simulink model "ES320A_MotDrvDiagc"  (R2013b)
settings: Solver=FixedStepDiscrete  StartTime=0.0  StopTime=1  FixedStep=.002  RelTol=1e-3
undefined symbols (not defined in the file): ARCHGLBPRM_2MILLISEC_SEC_F32, MotDrvDiagcErrFilFrq, MotDrvDiagcErrOffs, MotDrvDiagcErrThd, NtcNr1, NtcSts1, PHAONTISUMMAX_NANOSEC_U32, SysSt1
libraries: simulink x23, Fil x12, NxtrAbslt x6, NxtrLim x6
(part 1 of 3)
settings Model: Creator=PallavG  LastModifiedBy=FZG88Y
settings DataIOCC: LimitDataPoints=off  SaveFormat=Structure  ReturnWorkspaceOutputs=on
settings OptimizationCC: BlockReduction=off  InlineParams=on  ZeroExternalMemoryAtStartup=off  ZeroInternalMemoryAtStartup=off  OptimizeModelRefInitCode=on  LifeSpan=1
settings DebuggingCC: SignalInfNanChecking=error  SignalRangeChecking=warning  UnderspecifiedInitializationDetection=Simplified  SolverPrmCheckMsg=error  InheritedTsInSrcMsg=error  DiscreteInheritContinuousMsg=error  SingleTaskRateTransMsg=error  TasksWithSamePriorityMsg=error  SigSpecEnsureSampleTimeMsg=error  CheckMatrixSingularityMsg=error  IntegerOverflowMsg=error  ParameterUnderflowMsg=error  ParameterPrecisionLossMsg=error  ParameterTunabilityLossMsg=error  FixptConstUnderflowMsg=warning  FixptConstOverflowMsg=warning  VectorMatrixConversionMsg=error  SignalLabelMismatchMsg=error  UnconnectedInputMsg=error  UnconnectedOutputMsg=error  UnconnectedLineMsg=error  SFcnCompatibilityMsg=error  UniqueDataStoreMsg=warning  BusObjectLabelMismatch=error  RootOutportRequireBusObject=error  AssertControl=DisableAll  ModelReferenceIOMsg=error  ModelReferenceVersionMismatchMessage=warning  ModelReferenceIOMismatchMessage=error  ModelReferenceCSMismatchMessage=warning  ModelReferenceDataLoggingMessage=error  StateNameClashWarn=warning  StrictBusMsg=ErrorOnBusTreatedAsVector  NonBusSignalsTreatedAsBus=error  SFUnexpectedBacktrackingDiag=error  SFInvalidInputDataAccessInChartInitDiag=error  SFNoUnconditionalDefaultTransitionDiag=error  SFTransitionOutsideNaturalParentDiag=error  SFUnconditionalTransitionShadowingDiag=error  SFUndirectedBroadcastEventsDiag=error
settings ModelReferenceCC: ModelReferenceNumInstancesAllowed=Single
settings RTWCC: SystemTargetFile=autosar.tlc  GenCodeOnly=on  TemplateMakefile=ert_default_tmf  Description=AUTOSAR  GenerateReport=on  ProcessScript=autosar_make_rtw_hook  LaunchReport=on
settings CodeAppCC: GenerateComments=off  IgnoreCustomStorageClasses=off  CustomSymbolStrType=$N$R$M  CustomSymbolStrBlkIO=$N$M  SimulinkBlockComments=off
settings STFCustomTargetCC: ParMdlRefBuildCompliant=on  CompOptLevelCompliant=on  IncludeMdlTerminateFcn=off  CombineOutputUpdateFcns=on  SuppressErrorStatus=on  ERTFirstTimeCompliant=on  ERTCustomFileBanners=on  SupportNonFinite=off  SupportComplex=off  SupportContinuousTime=off  SupportNonInlinedSFcns=off  MATLABClassNameForMDSCustomization=Simulink.SoftwareTarget.ERTCustomization  AutosarCompliant=on  GRTInterface=off  SystemTargetFile=autosar.tlc
settings ERTTargetCC: CodeReplacementLibrary=ANSI_C  ConcurrentExecutionCompliant=off  IncludeMdlTerminateFcn=off  SuppressErrorStatus=on  SupportNonFinite=off  SupportComplex=off  ModelStepFunctionPrototypeControlCompliant=off  CPPClassGenCompliant=off  AutosarCompliant=on  InlinedParameterPlacement=NonHierarchical  ERTCustomFileTemplate=example_file_process.tlc  EnableUserReplacementTypes=on

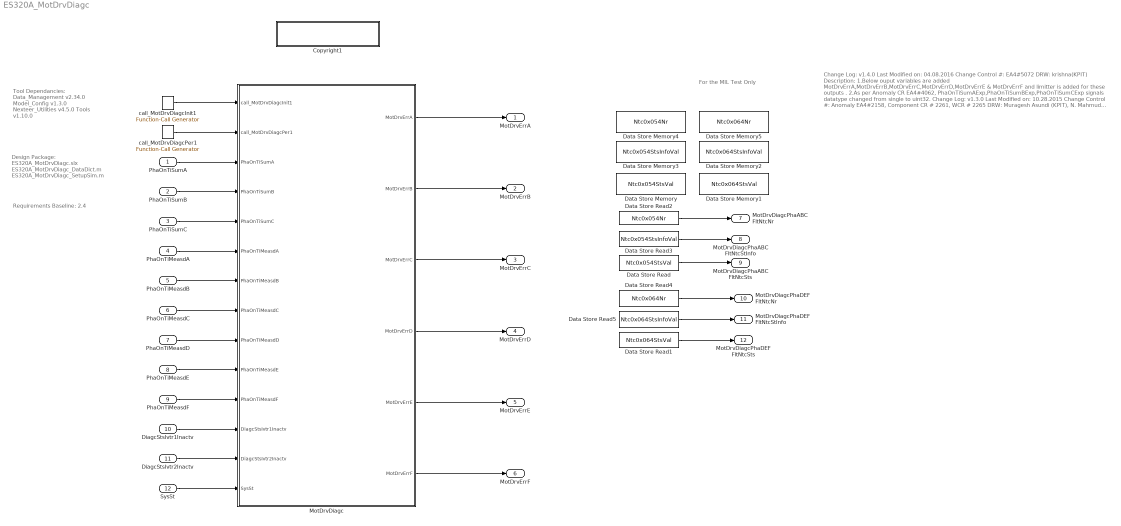
== system ES320A_MotDrvDiagc ==
  note: For the MIL Test Only
  note: Requirements Baseline: 2.4
  note: Design Package:
      | ES320A_MotDrvDiagc.slx
      | ES320A_MotDrvDiagc_DataDict.m
      | ES320A_MotDrvDiagc_SetupSim.m
  note: Change Log:  v1.4.0
      | Last Modified on: 04.08.2016
      | Change Control #: EA4#5072
      | DRW: krishna(KPIT)
      | Description:
      | 1.Below ouput variables are added
      |   MotDrvErrA,MotDrvErrB,MotDrvErrC,MotDrvErrD,MotDrvErrE & MotDrvErrF
      |   and limitter is added for these outputs .
      | 2.As per Anomaly CR EA4#4062, PhaOnTiSumAExp,PhaOnTiSumBExp,PhaOnTiSumCExp signals datatype
      | changed from single to uint32.
      |
      | Change Log:  v1.3.0
      | Last Modified on: 10.28.2015
      | Change Control #: Anomaly EA4#2158, Component CR # 2261, WCR # 2265
      | DRW:  Muragesh Asundi (KPIT), N. Mahmud
      | Description:
      | - Anomaly 2158 is fixed
      | - Also fixes the logic for setting the prepass, prefail for NTC54, 64
      |
      | Change Log:  v1.2.0
      | Last Modified on: 09.30.2015
      | Change Control #: Anomaly EA4#1595, Component CR # 1763, WCR # 1768
      | DRW:  N. Mahmud
      | Description:
      | - Anomaly 1595 is fixed
      |
      | Change Log:  v1.1.0
      | Date: 21-Aug-2015
      | Change Control #: EA4#1383
      | DRW:  Muragesh Asundi
      | Description:
      | - 'MotCtrl' prefix removed from Inputs.
      | - Global constant 'ARCHGLBPRM_2MILLISEC_SEC_F32' used
      |
      | Change Log:  v1.0.0
      | Date: 12-Aug-2015
      | Change Control #: EA4#1004
      | DRW:  Pallav Garg
      | Description:
      | - Initial Release of EA4 1.0.0
  note: Tool Dependancies:
      |
      | Data_Management v2.34.0
      | Model_Config v1.3.0
      | Nexteer_Utilities v4.5.0
      | Tools v1.10.0
  PhaOnTiSumA : Inport  RequirementInfo={'linktype_rmi_doors' '0000cf4c (/ESG Group/FDD Module Requirements/EA4 Specific/ES320A_MotDrvDiagc)' '#ES320A_92' 'true' 'REQ: ES320A_92' '' } %GIDa_5596e1da_8470_45ec_add7_471382801404
  PhaOnTiSumB : Inport  RequirementInfo={'linktype_rmi_doors' '0000cf4c (/ESG Group/FDD Module Requirements/EA4 Specific/ES320A_MotDrvDiagc)' '#ES320A_181' 'true' 'REQ: ES320A_181' '' } %GIDa_210e4004_e252_48ab_913f_51028c960f64  Port=2
  PhaOnTiSumC : Inport  RequirementInfo={'linktype_rmi_doors' '0000cf4c (/ESG Group/FDD Module Requirements/EA4 Specific/ES320A_MotDrvDiagc)' '#ES320A_180' 'true' 'REQ: ES320A_180' '' } %GIDa_70180edb_7662_4ea3_bdb5_76072d466fb3  Port=3
  PhaOnTiMeasdA : Inport  RequirementInfo={'linktype_rmi_doors' '0000cf4c (/ESG Group/FDD Module Requirements/EA4 Specific/ES320A_MotDrvDiagc)' '#ES320A_93' 'true' 'REQ: ES320A_93' '' } %GIDa_afd0493b_6092_46df_9f0f_5569d48d5c6b  Port=4
  PhaOnTiMeasdB : Inport  RequirementInfo={'linktype_rmi_doors' '0000cf4c (/ESG Group/FDD Module Requirements/EA4 Specific/ES320A_MotDrvDiagc)' '#ES320A_183' 'true' 'REQ: ES320A_183' '' } %GIDa_f1d745cb_f7fe_4c90_af22_8ff78fec897d  Port=5
  PhaOnTiMeasdC : Inport  RequirementInfo={'linktype_rmi_doors' '0000cf4c (/ESG Group/FDD Module Requirements/EA4 Specific/ES320A_MotDrvDiagc)' '#ES320A_182' 'true' 'REQ: ES320A_182' '' } %GIDa_39f5c4e7_f024_452a_b628_18bd5ec5a4db  Port=6
  PhaOnTiMeasdD : Inport  RequirementInfo={'linktype_rmi_doors' '0000cf4c (/ESG Group/FDD Module Requirements/EA4 Specific/ES320A_MotDrvDiagc)' '#ES320A_186' 'true' 'REQ: ES320A_186' '' } %GIDa_d08ff034_005a_421c_9828_e45c8ccc9891  Port=7
  PhaOnTiMeasdE : Inport  RequirementInfo={'linktype_rmi_doors' '0000cf4c (/ESG Group/FDD Module Requirements/EA4 Specific/ES320A_MotDrvDiagc)' '#ES320A_185' 'true' 'REQ: ES320A_185' '' } %GIDa_b8a159d2_0664_4d31_91d9_6025fe5fa159  Port=8
  PhaOnTiMeasdF : Inport  RequirementInfo={'linktype_rmi_doors' '0000cf4c (/ESG Group/FDD Module Requirements/EA4 Specific/ES320A_MotDrvDiagc)' '#ES320A_184' 'true' 'REQ: ES320A_184' '' } %GIDa_0e7ed425_9747_4174_868c_b8b73984cdca  Port=9
  DiagcStsIvtr1Inactv : Inport  RequirementInfo={'linktype_rmi_doors' '0000cf4c (/ESG Group/FDD Module Requirements/EA4 Specific/ES320A_MotDrvDiagc)' '#ES320A_187' 'true' 'REQ: ES320A_187' '' } %GIDa_a171dc8c_548f_4e98_b628_0ce941fa05d6  Port=10
  DiagcStsIvtr2Inactv : Inport  RequirementInfo={'linktype_rmi_doors' '0000cf4c (/ESG Group/FDD Module Requirements/EA4 Specific/ES320A_MotDrvDiagc)' '#ES320A_189' 'true' 'REQ: ES320A_189' '' } %GIDa_3630ab79_1ac9_45bf_b99f_436db09e5141  Port=11
  SysSt : Inport  RequirementInfo={'linktype_rmi_doors' '0000cf4c (/ESG Group/FDD Module Requirements/EA4 Specific/ES320A_MotDrvDiagc)' '#ES320A_188' 'true' 'REQ: ES320A_188' '' } %GIDa_0e538df3_d78e_40dd_9cd2_699620956152  Port=12
  Copyright1 : Subsystem  Description=|  RequirementInfo={} %GIDa_31a5e494_f362_4315_ad68_df9135c8582b  mask(Copyright Information){none=on}
      | Copyright info block.                                               
      |                                                                     
      | Place copyright information at the top of every subsystem in design.
      mask prompts: none "No parameters"
      mask help: Place copyright information at the top of every subsystem in design.
      mask Display:
      | NxtrConf = 'Nexteer Confidential';
      | 
      | sys = bdroot; %handle for the current model ("system")
      | first = get_param(sys,'Created');
      | if(isempty(first))
      |     first = datestr(now,'yyyy');
      | else
      |     first = first(end-3:end);  %year is last four digits
      | end
      | 
      | last = get_param(sys,'LastModifiedDate');
      | if isempty(last)
      |     last = datestr(now,'yyyy');
      | else
      |     last = last(end-3:end);
      | end
      | 
      | if strcmp(first,last)
      |     fprintf('%s\nCopyright  %s Nexteer',NxtrConf,first);
      | else
      |     fprintf('%s\n%s%s-%s Nexteer',NxtrConf,char(169),first,last);
      | end
  Data Store Read : DataStoreRead  DataStoreName=Ntc0x054StsVal  SampleTime=.002
  Data Store Read1 : DataStoreRead  DataStoreName=Ntc0x064StsVal  SampleTime=.002
  Data Store Read2 : DataStoreRead  DataStoreName=Ntc0x054Nr  SampleTime=.002
  Data Store Read3 : DataStoreRead  DataStoreName=Ntc0x054StsInfoVal  SampleTime=.002
  Data Store Read4 : DataStoreRead  DataStoreName=Ntc0x064Nr  SampleTime=.002
  Data Store Read5 : DataStoreRead  DataStoreName=Ntc0x064StsInfoVal  SampleTime=.002
  Data Store Memory : DataStoreMemory  DataStoreName=Ntc0x054StsVal  ReadBeforeWriteMsg=warning  WriteAfterWriteMsg=warning  WriteAfterReadMsg=warning  InitialValue=NtcSts1.NTCSTS_PASSD
  Data Store Memory1 : DataStoreMemory  DataStoreName=Ntc0x064StsVal  ReadBeforeWriteMsg=warning  WriteAfterWriteMsg=warning  WriteAfterReadMsg=warning  InitialValue=NtcSts1.NTCSTS_PASSD
  Data Store Memory2 : DataStoreMemory  DataStoreName=Ntc0x064StsInfoVal  ReadBeforeWriteMsg=warning  WriteAfterWriteMsg=warning  WriteAfterReadMsg=warning
  Data Store Memory3 : DataStoreMemory  DataStoreName=Ntc0x054StsInfoVal  ReadBeforeWriteMsg=warning  WriteAfterWriteMsg=warning  WriteAfterReadMsg=warning
  Data Store Memory4 : DataStoreMemory  DataStoreName=Ntc0x054Nr  ReadBeforeWriteMsg=warning  WriteAfterWriteMsg=warning  WriteAfterReadMsg=warning  InitialValue=NtcNr1.NTCNR_0X054
  Data Store Memory5 : DataStoreMemory  DataStoreName=Ntc0x064Nr  ReadBeforeWriteMsg=warning  WriteAfterWriteMsg=warning  WriteAfterReadMsg=warning  InitialValue=NtcNr1.NTCNR_0X064
  MotDrvDiagc : Subsystem
  call_MotDrvDiagcInit1 : simulink/Ports & Subsystems/Function-Call Generator  sample_time=.002  numberOfIterations=1
  call_MotDrvDiagcPer1 : simulink/Ports & Subsystems/Function-Call Generator  sample_time=.002  numberOfIterations=1
  MotDrvErrA : Outport
  MotDrvErrB : Outport  Port=2
  MotDrvErrC : Outport  Port=3
  MotDrvErrD : Outport  Port=4
  MotDrvErrE : Outport  Port=5
  MotDrvErrF : Outport  Port=6
  MotDrvDiagcPhaABCFltNtcNr : Outport  Port=7
  MotDrvDiagcPhaABCFltNtcStInfo : Outport  Port=8
  MotDrvDiagcPhaABCFltNtcSts : Outport  Port=9
  MotDrvDiagcPhaDEFFltNtcNr : Outport  Port=10
  MotDrvDiagcPhaDEFFltNtcStInfo : Outport  Port=11
  MotDrvDiagcPhaDEFFltNtcSts : Outport  Port=12
  wires:
  PhaOnTiSumA/1 -> MotDrvDiagc/3(PhaOnTiSumA)
  PhaOnTiSumB/1 -> MotDrvDiagc/4(PhaOnTiSumB)
  PhaOnTiSumC/1 -> MotDrvDiagc/5(PhaOnTiSumC)
  PhaOnTiMeasdA/1 -> MotDrvDiagc/6(PhaOnTiMeasdA)
  PhaOnTiMeasdB/1 -> MotDrvDiagc/7(PhaOnTiMeasdB)
  PhaOnTiMeasdC/1 -> MotDrvDiagc/8(PhaOnTiMeasdC)
  PhaOnTiMeasdD/1 -> MotDrvDiagc/9(PhaOnTiMeasdD)
  PhaOnTiMeasdE/1 -> MotDrvDiagc/10(PhaOnTiMeasdE)
  PhaOnTiMeasdF/1 -> MotDrvDiagc/11(PhaOnTiMeasdF)
  DiagcStsIvtr1Inactv/1 -> MotDrvDiagc/12(DiagcStsIvtr1Inactv)
  DiagcStsIvtr2Inactv/1 -> MotDrvDiagc/13(DiagcStsIvtr2Inactv)
  call_MotDrvDiagcPer1/1 -> MotDrvDiagc/2(call_MotDrvDiagcPer1)
  SysSt/1 -> MotDrvDiagc/14(SysSt)
  call_MotDrvDiagcInit1/1 -> MotDrvDiagc/1(call_MotDrvDiagcInit1)
  Data Store Read/1 -> MotDrvDiagcPhaABCFltNtcSts/1
  Data Store Read1/1 -> MotDrvDiagcPhaDEFFltNtcSts/1
  Data Store Read2/1 -> MotDrvDiagcPhaABCFltNtcNr/1
  Data Store Read3/1 -> MotDrvDiagcPhaABCFltNtcStInfo/1
  Data Store Read4/1 -> MotDrvDiagcPhaDEFFltNtcNr/1
  Data Store Read5/1 -> MotDrvDiagcPhaDEFFltNtcStInfo/1
  MotDrvDiagc/1(MotDrvErrA) -> MotDrvErrA/1
  MotDrvDiagc/2(MotDrvErrB) -> MotDrvErrB/1
  MotDrvDiagc/3(MotDrvErrC) -> MotDrvErrC/1
  MotDrvDiagc/6(MotDrvErrF) -> MotDrvErrF/1
  MotDrvDiagc/5(MotDrvErrE) -> MotDrvErrE/1
  MotDrvDiagc/4(MotDrvErrD) -> MotDrvErrD/1

== system ES320A_MotDrvDiagc/Copyright1 ==

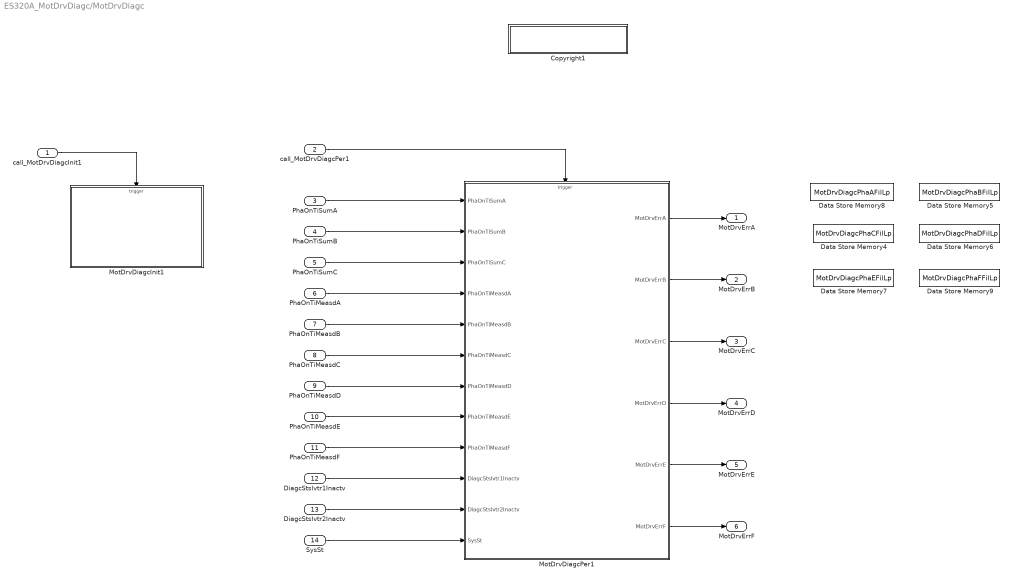
== system ES320A_MotDrvDiagc/MotDrvDiagc ==
  call_MotDrvDiagcInit1 : Inport
  call_MotDrvDiagcPer1 : Inport  Port=2
  PhaOnTiSumA : Inport  RequirementInfo={} %GIDa_46cfb15b_79f9_4df3_959a_549c348c89d2  Port=3
  PhaOnTiSumB : Inport  RequirementInfo="{}  %GIDa_e4750f2c_32c2_4abf_a78a_5be133e16fa3"  Port=4
  PhaOnTiSumC : Inport  Port=5
  PhaOnTiMeasdA : Inport  Port=6
  PhaOnTiMeasdB : Inport  Port=7
  PhaOnTiMeasdC : Inport  Port=8
  PhaOnTiMeasdD : Inport  Port=9
  PhaOnTiMeasdE : Inport  Port=10
  PhaOnTiMeasdF : Inport  Port=11
  DiagcStsIvtr1Inactv : Inport  Port=12
  DiagcStsIvtr2Inactv : Inport  Port=13
  SysSt : Inport  Port=14
  Copyright1 : Subsystem  Description=|  RequirementInfo={} %GIDa_40b2bef5_baed_40e1_9760_ec08ea904b84  mask(Copyright Information){none=on}
      | Copyright info block.                                               
      |                                                                     
      | Place copyright information at the top of every subsystem in design.
      mask prompts: none "No parameters"
      mask help: Place copyright information at the top of every subsystem in design.
      mask Display:
      | NxtrConf = 'Nexteer Confidential';
      | 
      | sys = bdroot; %handle for the current model ("system")
      | first = get_param(sys,'Created');
      | if(isempty(first))
      |     first = datestr(now,'yyyy');
      | else
      |     first = first(end-3:end);  %year is last four digits
      | end
      | 
      | last = get_param(sys,'LastModifiedDate');
      | if isempty(last)
      |     last = datestr(now,'yyyy');
      | else
      |     last = last(end-3:end);
      | end
      | 
      | if strcmp(first,last)
      |     fprintf('%s\nCopyright  %s Nexteer',NxtrConf,first);
      | else
      |     fprintf('%s\n%s%s-%s Nexteer',NxtrConf,char(169),first,last);
      | end
  Data Store Memory4 : DataStoreMemory  DataStoreName=MotDrvDiagcPhaCFilLp  InitialValue=struct('FilSt',single(0),'FilGain',single(0))  OutDataTypeStr=Bus: FilLpRec1  StateMustResolveToSignalObject=on
  Data Store Memory5 : DataStoreMemory  DataStoreName=MotDrvDiagcPhaBFilLp  InitialValue=struct('FilSt',single(0),'FilGain',single(0))  OutDataTypeStr=Bus: FilLpRec1  StateMustResolveToSignalObject=on
  Data Store Memory6 : DataStoreMemory  DataStoreName=MotDrvDiagcPhaDFilLp  InitialValue=struct('FilSt',single(0),'FilGain',single(0))  OutDataTypeStr=Bus: FilLpRec1  StateMustResolveToSignalObject=on
  Data Store Memory7 : DataStoreMemory  DataStoreName=MotDrvDiagcPhaEFilLp  InitialValue=struct('FilSt',single(0),'FilGain',single(0))  OutDataTypeStr=Bus: FilLpRec1  StateMustResolveToSignalObject=on
  Data Store Memory8 : DataStoreMemory  DataStoreName=MotDrvDiagcPhaAFilLp  InitialValue=struct('FilSt',single(0),'FilGain',single(0))  OutDataTypeStr=Bus: FilLpRec1  StateMustResolveToSignalObject=on
  Data Store Memory9 : DataStoreMemory  DataStoreName=MotDrvDiagcPhaFFilLp  InitialValue=struct('FilSt',single(0),'FilGain',single(0))  OutDataTypeStr=Bus: FilLpRec1  StateMustResolveToSignalObject=on
  MotDrvDiagcInit1 : Subsystem
  MotDrvDiagcPer1 : Subsystem  RequirementInfo={'linktype_rmi_doors' '0000cf4c (/ESG Group/FDD Module Requirements/EA4 Specific/ES320A_MotDrvDiagc)' '#ES320A_158' 'true' 'REQ: ES320A_158' '' ; 'linktype_rmi_doors' '0000cf4c (/ESG Group/FDD Module Requirements/EA4 Specific/ES320A_MotDrvDiagc)' '#ES320A_160' 'true' 'REQ: ES320A_160' '' } %GIDa_e8681813_4efe_4d27_b36c_1f578861e450
  MotDrvErrA : Outport  RequirementInfo={'linktype_rmi_doors' '0000cf4c (/ESG Group/FDD Module Requirements/EA4 Specific/ES320A_MotDrvDiagc)' '#ES320A_207' 'true' 'REQ: ES320A_207' '' } %GIDa_9503e4c0_a7fc_485b_98a2_972c7f7bfe08
  MotDrvErrB : Outport  RequirementInfo={'linktype_rmi_doors' '0000cf4c (/ESG Group/FDD Module Requirements/EA4 Specific/ES320A_MotDrvDiagc)' '#ES320A_207' 'true' 'REQ: ES320A_207' '' } %GIDa_84eb9338_eb0d_4322_a092_261cb67f10b3  Port=2
  MotDrvErrC : Outport  RequirementInfo={'linktype_rmi_doors' '0000cf4c (/ESG Group/FDD Module Requirements/EA4 Specific/ES320A_MotDrvDiagc)' '#ES320A_206' 'true' 'REQ: ES320A_206' '' } %GIDa_9cdd7cca_5e7a_4907_9b10_5ffe4d089f88  Port=3
  MotDrvErrD : Outport  RequirementInfo={'linktype_rmi_doors' '0000cf4c (/ESG Group/FDD Module Requirements/EA4 Specific/ES320A_MotDrvDiagc)' '#ES320A_205' 'true' 'REQ: ES320A_205' '' } %GIDa_f1a02c70_5322_40ef_93da_787d66763215  Port=4
  MotDrvErrE : Outport  RequirementInfo={'linktype_rmi_doors' '0000cf4c (/ESG Group/FDD Module Requirements/EA4 Specific/ES320A_MotDrvDiagc)' '#ES320A_204' 'true' 'REQ: ES320A_204' '' } %GIDa_72a22f43_ae99_4136_a3a8_5e5738f24507  Port=5
  MotDrvErrF : Outport  RequirementInfo={'linktype_rmi_doors' '0000cf4c (/ESG Group/FDD Module Requirements/EA4 Specific/ES320A_MotDrvDiagc)' '#ES320A_203' 'true' 'REQ: ES320A_203' '' } %GIDa_ddfd7e60_4b6a_46f1_bcfa_2573913685dc  Port=6
  wires:
  PhaOnTiMeasdC/1 -> MotDrvDiagcPer1/6(PhaOnTiMeasdC)
  PhaOnTiMeasdD/1 -> MotDrvDiagcPer1/7(PhaOnTiMeasdD)
  PhaOnTiSumB/1 -> MotDrvDiagcPer1/2(PhaOnTiSumB)
  PhaOnTiMeasdE/1 -> MotDrvDiagcPer1/8(PhaOnTiMeasdE)
  PhaOnTiMeasdF/1 -> MotDrvDiagcPer1/9(PhaOnTiMeasdF)
  PhaOnTiSumC/1 -> MotDrvDiagcPer1/3(PhaOnTiSumC)
  DiagcStsIvtr1Inactv/1 -> MotDrvDiagcPer1/10(DiagcStsIvtr1Inactv)
  DiagcStsIvtr2Inactv/1 -> MotDrvDiagcPer1/11(DiagcStsIvtr2Inactv)
  call_MotDrvDiagcPer1/1 -> MotDrvDiagcPer1/Trigger
  SysSt/1 -> MotDrvDiagcPer1/12(SysSt)
  call_MotDrvDiagcInit1/1 -> MotDrvDiagcInit1/Trigger
  PhaOnTiSumA/1 -> MotDrvDiagcPer1/1(PhaOnTiSumA)
  MotDrvDiagcPer1/1(MotDrvErrA) -> MotDrvErrA/1
  MotDrvDiagcPer1/2(MotDrvErrB) -> MotDrvErrB/1
  MotDrvDiagcPer1/3(MotDrvErrC) -> MotDrvErrC/1
  MotDrvDiagcPer1/4(MotDrvErrD) -> MotDrvErrD/1
  MotDrvDiagcPer1/5(MotDrvErrE) -> MotDrvErrE/1
  MotDrvDiagcPer1/6(MotDrvErrF) -> MotDrvErrF/1
  PhaOnTiMeasdA/1 -> MotDrvDiagcPer1/4(PhaOnTiMeasdA)
  PhaOnTiMeasdB/1 -> MotDrvDiagcPer1/5(PhaOnTiMeasdB)

== system ES320A_MotDrvDiagc/MotDrvDiagc/Copyright1 ==

== system ES320A_MotDrvDiagc/MotDrvDiagc/MotDrvDiagcInit1 ==
  function : TriggerPort  TriggerType=function-call
  Copyright1 : Subsystem  Description=|  RequirementInfo={} %GIDa_0a1cd7fa_88a7_493f_9ffa_3855db88fd16  mask(Copyright Information){none=on}
      | Copyright info block.                                               
      |                                                                     
      | Place copyright information at the top of every subsystem in design.
      mask prompts: none "No parameters"
      mask help: Place copyright information at the top of every subsystem in design.
      mask Display:
      | NxtrConf = 'Nexteer Confidential';
      | 
      | sys = bdroot; %handle for the current model ("system")
      | first = get_param(sys,'Created');
      | if(isempty(first))
      |     first = datestr(now,'yyyy');
      | else
      |     first = first(end-3:end);  %year is last four digits
      | end
      | 
      | last = get_param(sys,'LastModifiedDate');
      | if isempty(last)
      |     last = datestr(now,'yyyy');
      | else
      |     last = last(end-3:end);
      | end
      | 
      | if strcmp(first,last)
      |     fprintf('%s\nCopyright  %s Nexteer',NxtrConf,first);
      | else
      |     fprintf('%s\n%s%s-%s Nexteer',NxtrConf,char(169),first,last);
      | end
  MotDrvDiagcPhaAFilLpInit : Fil/FilLpInit  Ic=0  Ts=ARCHGLBPRM_2MILLISEC_SEC_F32  Freq=MotDrvDiagcErrFilFrq  StVar=MotDrvDiagcPhaAFilLp
  MotDrvDiagcPhaBFilLpInit : Fil/FilLpInit  Ic=0  Ts=ARCHGLBPRM_2MILLISEC_SEC_F32  Freq=MotDrvDiagcErrFilFrq  StVar=MotDrvDiagcPhaBFilLp
  MotDrvDiagcPhaCFilLpInit : Fil/FilLpInit  Ic=0  Ts=ARCHGLBPRM_2MILLISEC_SEC_F32  Freq=MotDrvDiagcErrFilFrq  StVar=MotDrvDiagcPhaCFilLp
  MotDrvDiagcPhaDFilLpInit : Fil/FilLpInit  Ic=0  Ts=ARCHGLBPRM_2MILLISEC_SEC_F32  Freq=MotDrvDiagcErrFilFrq  StVar=MotDrvDiagcPhaDFilLp
  MotDrvDiagcPhaEFilLpInit : Subsystem  AncestorBlock=Fil/FilLpInit  mask(FilLpInit){Ic=0, Ts=ARCHGLBPRM_2MILLISEC_SEC_F32, Freq=MotDrvDiagcErrFilFrq, StVar=MotDrvDiagcPhaEFilLp}
      mask prompts: Ic "Initial Value"; Ts "TimeStep:"; Freq "Frequency:"; StVar "State Variable"
      mask init:
      | blk = gcb;
      | set_param([blk '/FilLpUpdGain'],'Ts',Ts)
      | set_param([blk '/FilLpUpdGain'],'StVar',StVar)
      | set_param([blk '/Freq'],'Value',Freq)
      | set_param([blk '/Ic'],'Value',Ic)
      | set_param([ blk '/Data Store Write'],'DataStoreName',StVar)
      | try
      |     dt = evalin('base',[StVar '.EngDT']);
      | catch err
      |     if strcmp(err.identifier,'MATLAB:undefinedVarOrClass')
      |         dt = struct.FilLpRec1;
      |     end
      | end
      | if isa(dt,'struct.FilLpRec1')
      | set_param([ blk '/Data Store Write'],'DataStoreElements',[StVar '.FilGain'])
      | elseif isa(dt,'struct.FilHpRec1')
      | set_param([ blk '/Data Store Write'],'DataStoreElements',[StVar '.FilLpRec.FilGain'])
      | else
      |     error('Incorrect data class.');
      | end
      mask Display:
      | text(0.35,0.9,'FilLpInit')
      | text(0.05,0.7,['Ic: ' Ic])
      | text(0.05,0.5,['Ts: ' Ts])
      | text(0.05,0.3,['Freq: ' Freq])
      | text(0.05,0.1,['StVar: ' StVar])
  MotDrvDiagcPhaFFilLpInit : Subsystem  AncestorBlock=Fil/FilLpInit  mask(FilLpInit){Ic=0, Ts=ARCHGLBPRM_2MILLISEC_SEC_F32, Freq=MotDrvDiagcErrFilFrq, StVar=MotDrvDiagcPhaFFilLp}
      mask prompts: Ic "Initial Value"; Ts "TimeStep:"; Freq "Frequency:"; StVar "State Variable"
      mask init: same as ES320A_MotDrvDiagc/MotDrvDiagc/MotDrvDiagcInit1/MotDrvDiagcPhaEFilLpInit
      mask Display:
      | text(0.35,0.9,'FilLpInit')
      | text(0.05,0.7,['Ic: ' Ic])
      | text(0.05,0.5,['Ts: ' Ts])
      | text(0.05,0.3,['Freq: ' Freq])
      | text(0.05,0.1,['StVar: ' StVar])

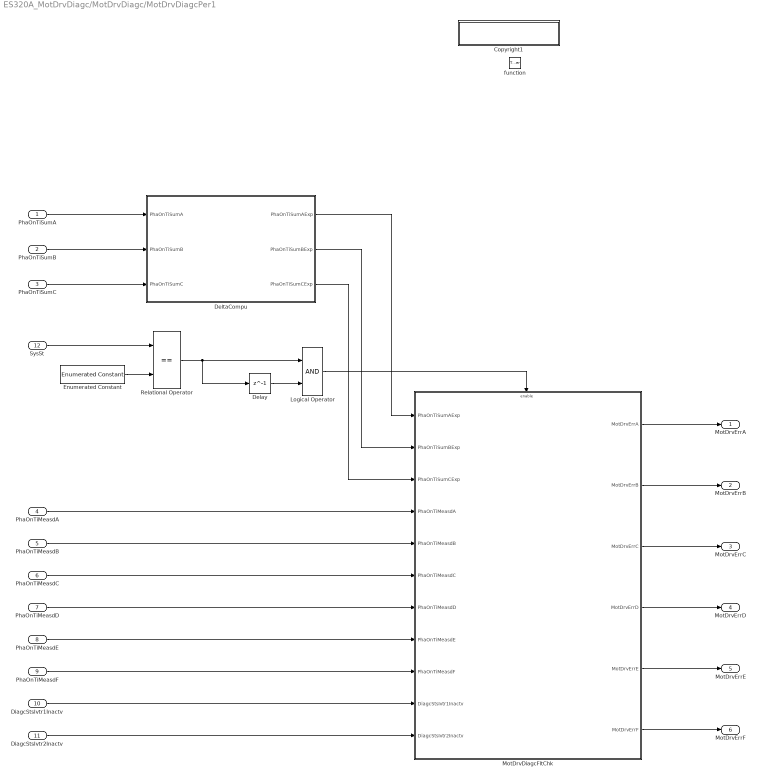
== system ES320A_MotDrvDiagc/MotDrvDiagc/MotDrvDiagcPer1 ==
  PhaOnTiSumA : Inport
  PhaOnTiSumB : Inport  Port=2
  PhaOnTiSumC : Inport  Port=3
  PhaOnTiMeasdA : Inport  Port=4
  PhaOnTiMeasdB : Inport  Port=5
  PhaOnTiMeasdC : Inport  Port=6
  PhaOnTiMeasdD : Inport  Port=7
  PhaOnTiMeasdE : Inport  Port=8
  PhaOnTiMeasdF : Inport  Port=9
  DiagcStsIvtr1Inactv : Inport  Port=10
  DiagcStsIvtr2Inactv : Inport  Port=11
  SysSt : Inport  Port=12  OutDataTypeStr=Enum: SysSt1
  function : TriggerPort  TriggerType=function-call
  Copyright1 : Subsystem  Description=|  RequirementInfo={} %GIDa_b6a8f04b_092f_4b64_aeb7_200da596c9ae  mask(Copyright Information){none=on}
      | Copyright info block.                                               
      |                                                                     
      | Place copyright information at the top of every subsystem in design.
      mask prompts: none "No parameters"
      mask help: Place copyright information at the top of every subsystem in design.
      mask Display:
      | NxtrConf = 'Nexteer Confidential';
      | 
      | sys = bdroot; %handle for the current model ("system")
      | first = get_param(sys,'Created');
      | if(isempty(first))
      |     first = datestr(now,'yyyy');
      | else
      |     first = first(end-3:end);  %year is last four digits
      | end
      | 
      | last = get_param(sys,'LastModifiedDate');
      | if isempty(last)
      |     last = datestr(now,'yyyy');
      | else
      |     last = last(end-3:end);
      | end
      | 
      | if strcmp(first,last)
      |     fprintf('%s\nCopyright  %s Nexteer',NxtrConf,first);
      | else
      |     fprintf('%s\n%s%s-%s Nexteer',NxtrConf,char(169),first,last);
      | end
  Delay : Delay  DelayLength=1  InitialCondition=0  StateName=UnitDly
  DeltaCompu : Subsystem
  Enumerated Constant : simulink/Sources/Enumerated Constant  OutDataTypeStr=Enum: SysSt1  Value=SysSt1.SYSST_ENA  SampleTime=inf
  Logical Operator : Logic  AllPortsSameDT=off  OutDataTypeStr=boolean
  MotDrvDiagcFltChk : Subsystem
  Relational Operator : RelationalOperator  Operator===  OutDataTypeStr=boolean
  MotDrvErrA : Outport
  MotDrvErrB : Outport  Port=2
  MotDrvErrC : Outport  Port=3
  MotDrvErrD : Outport  Port=4
  MotDrvErrE : Outport  Port=5
  MotDrvErrF : Outport  Port=6
  wires:
  PhaOnTiMeasdA/1 -> MotDrvDiagcFltChk/4(PhaOnTiMeasdA)
  PhaOnTiMeasdB/1 -> MotDrvDiagcFltChk/5(PhaOnTiMeasdB)
  PhaOnTiMeasdC/1 -> MotDrvDiagcFltChk/6(PhaOnTiMeasdC)
  PhaOnTiMeasdD/1 -> MotDrvDiagcFltChk/7(PhaOnTiMeasdD)
  PhaOnTiMeasdE/1 -> MotDrvDiagcFltChk/8(PhaOnTiMeasdE)
  PhaOnTiMeasdF/1 -> MotDrvDiagcFltChk/9(PhaOnTiMeasdF)
  DiagcStsIvtr1Inactv/1 -> MotDrvDiagcFltChk/10(DiagcStsIvtr1Inactv)
  DiagcStsIvtr2Inactv/1 -> MotDrvDiagcFltChk/11(DiagcStsIvtr2Inactv)
  Logical Operator/1 -> MotDrvDiagcFltChk/Enable
  SysSt/1 -> Relational Operator/1
  Enumerated Constant/1 -> Relational Operator/2
  PhaOnTiSumC/1 -> DeltaCompu/3(PhaOnTiSumC)
  PhaOnTiSumB/1 -> DeltaCompu/2(PhaOnTiSumB)
  DeltaCompu/1(PhaOnTiSumAExp) -> MotDrvDiagcFltChk/1(PhaOnTiSumAExp)
  DeltaCompu/2(PhaOnTiSumBExp) -> MotDrvDiagcFltChk/2(PhaOnTiSumBExp)
  DeltaCompu/3(PhaOnTiSumCExp) -> MotDrvDiagcFltChk/3(PhaOnTiSumCExp)
  PhaOnTiSumA/1 -> DeltaCompu/1(PhaOnTiSumA)
  Delay/1 -> Logical Operator/2
  Relational Operator/1 -> Delay/1, Logical Operator/1
  MotDrvDiagcFltChk/1(MotDrvErrA) -> MotDrvErrA/1
  MotDrvDiagcFltChk/2(MotDrvErrB) -> MotDrvErrB/1
  MotDrvDiagcFltChk/3(MotDrvErrC) -> MotDrvErrC/1
  MotDrvDiagcFltChk/5(MotDrvErrE) -> MotDrvErrE/1
  MotDrvDiagcFltChk/4(MotDrvErrD) -> MotDrvErrD/1
  MotDrvDiagcFltChk/6(MotDrvErrF) -> MotDrvErrF/1

== system ES320A_MotDrvDiagc/MotDrvDiagc/MotDrvDiagcInit1/Copyright1 ==

== system ES320A_MotDrvDiagc/MotDrvDiagc/MotDrvDiagcInit1/MotDrvDiagcPhaEFilLpInit ==
  Data Store Write : DataStoreWrite  DataStoreName=MotDrvDiagcPhaEFilLp  DataStoreElements=MotDrvDiagcPhaEFilLp.FilGain
  FilLpUpdGain : Fil/FilLpUpdGain  Ts=ARCHGLBPRM_2MILLISEC_SEC_F32  StVar=MotDrvDiagcPhaEFilLp
  Freq : Constant  Value=MotDrvDiagcErrFilFrq  OutDataTypeStr=single
  Ic : Constant  Value=0  OutDataTypeStr=single
  wires:
  Ic/1 -> Data Store Write/1
  Freq/1 -> FilLpUpdGain/1

== system ES320A_MotDrvDiagc/MotDrvDiagc/MotDrvDiagcInit1/MotDrvDiagcPhaFFilLpInit ==
  Data Store Write : DataStoreWrite  DataStoreName=MotDrvDiagcPhaFFilLp  DataStoreElements=MotDrvDiagcPhaFFilLp.FilGain
  FilLpUpdGain : Fil/FilLpUpdGain  Ts=ARCHGLBPRM_2MILLISEC_SEC_F32  StVar=MotDrvDiagcPhaFFilLp
  Freq : Constant  Value=MotDrvDiagcErrFilFrq  OutDataTypeStr=single
  Ic : Constant  Value=0  OutDataTypeStr=single
  wires:
  Ic/1 -> Data Store Write/1
  Freq/1 -> FilLpUpdGain/1

== system ES320A_MotDrvDiagc/MotDrvDiagc/MotDrvDiagcPer1/Copyright1 ==

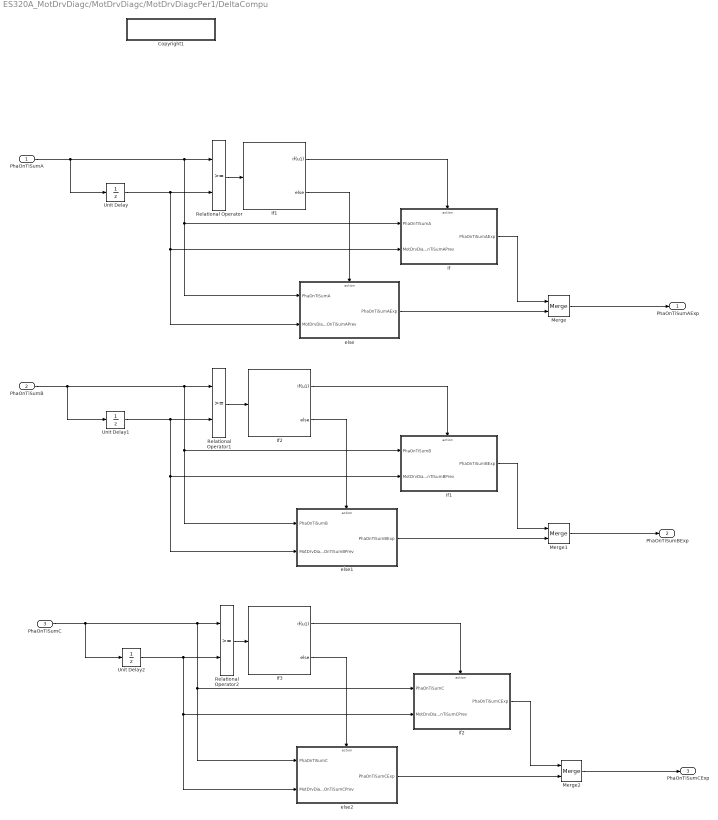
== system ES320A_MotDrvDiagc/MotDrvDiagc/MotDrvDiagcPer1/DeltaCompu ==
  PhaOnTiSumA : Inport
  PhaOnTiSumB : Inport  Port=2
  PhaOnTiSumC : Inport  Port=3
  Copyright1 : Subsystem  Description=|  RequirementInfo={} %GIDa_601d2834_462b_4532_b5dc_96903db13663  mask(Copyright Information){none=on}
      | Copyright info block.                                               
      |                                                                     
      | Place copyright information at the top of every subsystem in design.
      mask prompts: none "No parameters"
      mask help: Place copyright information at the top of every subsystem in design.
      mask Display:
      | NxtrConf = 'Nexteer Confidential';
      | 
      | sys = bdroot; %handle for the current model ("system")
      | first = get_param(sys,'Created');
      | if(isempty(first))
      |     first = datestr(now,'yyyy');
      | else
      |     first = first(end-3:end);  %year is last four digits
      | end
      | 
      | last = get_param(sys,'LastModifiedDate');
      | if isempty(last)
      |     last = datestr(now,'yyyy');
      | else
      |     last = last(end-3:end);
      | end
      | 
      | if strcmp(first,last)
      |     fprintf('%s\nCopyright  %s Nexteer',NxtrConf,first);
      | else
      |     fprintf('%s\n%s%s-%s Nexteer',NxtrConf,char(169),first,last);
      | end
  If1 : If  RequirementInfo={} %GIDa_ea6a79cb_0936_420c_8ede_b02280241c5d  IfExpression=u1
  If2 : If  RequirementInfo={} %GIDa_0014b097_5cca_4ec6_8fb8_db8d9e19247e  IfExpression=u1
  If3 : If  RequirementInfo={} %GIDa_cb8298b6_3a53_4d78_8774_1471c8816162  IfExpression=u1
  Merge : Merge
  Merge1 : Merge
  Merge2 : Merge
  Relational Operator : RelationalOperator  OutDataTypeStr=boolean
  Relational Operator1 : RelationalOperator  OutDataTypeStr=boolean
  Relational Operator2 : RelationalOperator  OutDataTypeStr=boolean
  Unit Delay : UnitDelay  SampleTime=-1  StateName=MotDrvDiagcPhaOnTiSumAPrev  StateMustResolveToSignalObject=on
      settings: AttributesFormatString=MotDrvDiagcPhaOnTiSumAPrev
  Unit Delay1 : UnitDelay  SampleTime=-1  StateName=MotDrvDiagcPhaOnTiSumBPrev  StateMustResolveToSignalObject=on
      settings: AttributesFormatString=MotDrvDiagcPhaOnTiSumBPrev
  Unit Delay2 : UnitDelay  SampleTime=-1  StateName=MotDrvDiagcPhaOnTiSumCPrev  StateMustResolveToSignalObject=on
      settings: AttributesFormatString=MotDrvDiagcPhaOnTiSumCPrev
  else : Subsystem
  else1 : Subsystem
  else2 : Subsystem
  if : Subsystem  RequirementInfo={} %GIDa_34f2964d_b23e_455c_bb42_472f7a311333
  if1 : Subsystem  RequirementInfo={} %GIDa_8bb4ca3d_c102_4af0_8f7e_d8f0042659f7
  if2 : Subsystem  RequirementInfo={} %GIDa_1678200f_e622_44c6_a191_d3be54666f2c
  PhaOnTiSumAExp : Outport
  PhaOnTiSumBExp : Outport  Port=2
  PhaOnTiSumCExp : Outport  Port=3
  wires:
  PhaOnTiSumA/1 -> Unit Delay/1, Relational Operator/1, if/1(PhaOnTiSumA), else/1(PhaOnTiSumA)
  Unit Delay/1 -> Relational Operator/2, if/2(MotDrvDiagcPhaOnTiSumAPrev), else/2(MotDrvDiagcPhaOnTiSumAPrev)
  If1/1 -> if/Action
  If1/2 -> else/Action
  if/1(PhaOnTiSumAExp) -> Merge/1
  else/1(PhaOnTiSumAExp) -> Merge/2
  PhaOnTiSumB/1 -> Unit Delay1/1, Relational Operator1/1, if1/1(PhaOnTiSumB), else1/1(PhaOnTiSumB)
  Unit Delay1/1 -> Relational Operator1/2, if1/2(MotDrvDiagcPhaOnTiSumBPrev), else1/2(MotDrvDiagcPhaOnTiSumBPrev)
  If2/1 -> if1/Action
  If2/2 -> else1/Action
  if1/1(PhaOnTiSumBExp) -> Merge1/1
  else1/1(PhaOnTiSumBExp) -> Merge1/2
  PhaOnTiSumC/1 -> Relational Operator2/1, if2/1(PhaOnTiSumC), else2/1(PhaOnTiSumC), Unit Delay2/1
  Unit Delay2/1 -> Relational Operator2/2, if2/2(MotDrvDiagcPhaOnTiSumCPrev), else2/2(MotDrvDiagcPhaOnTiSumCPrev)
  If3/1 -> if2/Action
  If3/2 -> else2/Action
  if2/1(PhaOnTiSumCExp) -> Merge2/1
  else2/1(PhaOnTiSumCExp) -> Merge2/2
  Relational Operator/1 -> If1/1
  Relational Operator1/1 -> If2/1
  Relational Operator2/1 -> If3/1
  Merge1/1 -> PhaOnTiSumBExp/1
  Merge2/1 -> PhaOnTiSumCExp/1
  Merge/1 -> PhaOnTiSumAExp/1

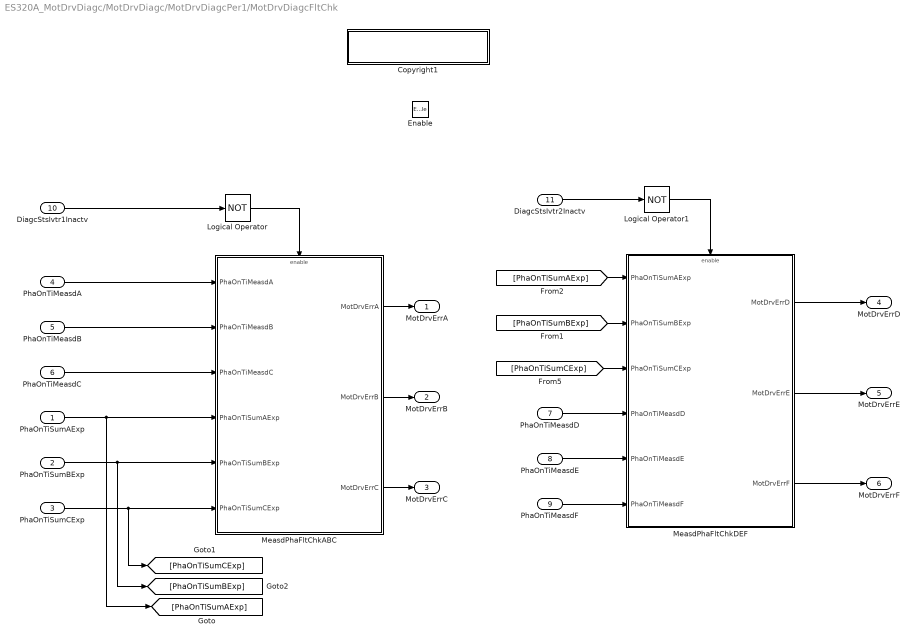
== system ES320A_MotDrvDiagc/MotDrvDiagc/MotDrvDiagcPer1/MotDrvDiagcFltChk ==
  PhaOnTiSumAExp : Inport
  PhaOnTiSumBExp : Inport  Port=2
  PhaOnTiSumCExp : Inport  Port=3
  PhaOnTiMeasdA : Inport  Port=4
  PhaOnTiMeasdB : Inport  Port=5
  PhaOnTiMeasdC : Inport  Port=6
  PhaOnTiMeasdD : Inport  Port=7
  PhaOnTiMeasdE : Inport  Port=8
  PhaOnTiMeasdF : Inport  Port=9
  DiagcStsIvtr1Inactv : Inport  Port=10
  DiagcStsIvtr2Inactv : Inport  Port=11
  Enable : EnablePort  StatesWhenEnabling=reset
  Copyright1 : Subsystem  Description=|  RequirementInfo={} %GIDa_0dc7ab09_e3ae_4417_8a5d_58e410e0a101  mask(Copyright Information){none=on}
      | Copyright info block.                                               
      |                                                                     
      | Place copyright information at the top of every subsystem in design.
      mask prompts: none "No parameters"
      mask help: Place copyright information at the top of every subsystem in design.
      mask Display:
      | NxtrConf = 'Nexteer Confidential';
      | 
      | sys = bdroot; %handle for the current model ("system")
      | first = get_param(sys,'Created');
      | if(isempty(first))
      |     first = datestr(now,'yyyy');
      | else
      |     first = first(end-3:end);  %year is last four digits
      | end
      | 
      | last = get_param(sys,'LastModifiedDate');
      | if isempty(last)
      |     last = datestr(now,'yyyy');
      | else
      |     last = last(end-3:end);
      | end
      | 
      | if strcmp(first,last)
      |     fprintf('%s\nCopyright  %s Nexteer',NxtrConf,first);
      | else
      |     fprintf('%s\n%s%s-%s Nexteer',NxtrConf,char(169),first,last);
      | end
  Logical Operator : Logic  Operator=NOT  AllPortsSameDT=off  OutDataTypeStr=boolean
  Logical Operator1 : Logic  Operator=NOT  AllPortsSameDT=off  OutDataTypeStr=boolean
  MeasdPhaFltChkABC : Subsystem  RequirementInfo={'linktype_rmi_doors' '0000cf4c (/ESG Group/FDD Module Requirements/EA4 Specific/ES320A_MotDrvDiagc)' '#ES320A_29' 'true' 'REQ: ES320A_29' '' ; 'linktype_rmi_doors' '0000cf4c (/ESG Group/FDD Module Requirements/EA4 Specific/ES320A_MotDrvDiagc)' '#ES320A_144' 'true' 'REQ: ES320A_144' '' ; 'linktype_rmi_doors' '0000cf4c (/ESG Group/FDD Module Requirements/EA4 Specific/ES320A_MotDrvDiagc)' '#ES320A_104' 'true' 'REQ: ES320A_104' '' } %GIDa_5af5cf17_7156_4b05_96ca_f5e6f025f324
  MeasdPhaFltChkDEF : Subsystem  RequirementInfo={'linktype_rmi_doors' '0000cf4c (/ESG Group/FDD Module Requirements/EA4 Specific/ES320A_MotDrvDiagc)' '#ES320A_29' 'true' 'REQ: ES320A_29' '' ; 'linktype_rmi_doors' '0000cf4c (/ESG Group/FDD Module Requirements/EA4 Specific/ES320A_MotDrvDiagc)' '#ES320A_144' 'true' 'REQ: ES320A_144' '' ; 'linktype_rmi_doors' '0000cf4c (/ESG Group/FDD Module Requirements/EA4 Specific/ES320A_MotDrvDiagc)' '#ES320A_104' 'true' 'REQ: ES320A_104' '' } %GIDa_de7cebe5_42eb_45b7_9860_074335d663ba
  MotDrvErrA : Outport
  MotDrvErrB : Outport  Port=2
  MotDrvErrC : Outport  Port=3
  MotDrvErrD : Outport  Port=4
  MotDrvErrE : Outport  Port=5
  MotDrvErrF : Outport  Port=6
  wires:
  PhaOnTiMeasdA/1 -> MeasdPhaFltChkABC/1(PhaOnTiMeasdA)
  PhaOnTiMeasdC/1 -> MeasdPhaFltChkABC/3(PhaOnTiMeasdC)
  PhaOnTiMeasdB/1 -> MeasdPhaFltChkABC/2(PhaOnTiMeasdB)
  DiagcStsIvtr1Inactv/1 -> Logical Operator/1
  DiagcStsIvtr2Inactv/1 -> Logical Operator1/1
  PhaOnTiSumAExp/1 -> MeasdPhaFltChkABC/4(PhaOnTiSumAExp), [PhaOnTiSumAExp]
  PhaOnTiSumCExp/1 -> MeasdPhaFltChkABC/6(PhaOnTiSumCExp), [PhaOnTiSumCExp]
  PhaOnTiSumBExp/1 -> MeasdPhaFltChkABC/5(PhaOnTiSumBExp), [PhaOnTiSumBExp]
  [PhaOnTiSumBExp] -> MeasdPhaFltChkDEF/2(PhaOnTiSumBExp)
  Logical Operator/1 -> MeasdPhaFltChkABC/Enable
  Logical Operator1/1 -> MeasdPhaFltChkDEF/Enable
  [PhaOnTiSumAExp] -> MeasdPhaFltChkDEF/1(PhaOnTiSumAExp)
  [PhaOnTiSumCExp] -> MeasdPhaFltChkDEF/3(PhaOnTiSumCExp)
  PhaOnTiMeasdD/1 -> MeasdPhaFltChkDEF/4(PhaOnTiMeasdD)
  PhaOnTiMeasdE/1 -> MeasdPhaFltChkDEF/5(PhaOnTiMeasdE)
  PhaOnTiMeasdF/1 -> MeasdPhaFltChkDEF/6(PhaOnTiMeasdF)
  MeasdPhaFltChkABC/3(MotDrvErrC) -> MotDrvErrC/1
  MeasdPhaFltChkABC/2(MotDrvErrB) -> MotDrvErrB/1
  MeasdPhaFltChkABC/1(MotDrvErrA) -> MotDrvErrA/1
  MeasdPhaFltChkDEF/1(MotDrvErrD) -> MotDrvErrD/1
  MeasdPhaFltChkDEF/2(MotDrvErrE) -> MotDrvErrE/1
  MeasdPhaFltChkDEF/3(MotDrvErrF) -> MotDrvErrF/1

== system ES320A_MotDrvDiagc/MotDrvDiagc/MotDrvDiagcPer1/DeltaCompu/Copyright1 ==

== system ES320A_MotDrvDiagc/MotDrvDiagc/MotDrvDiagcPer1/DeltaCompu/else ==
  PhaOnTiSumA : Inport
  MotDrvDiagcPhaOnTiSumAPrev : Inport  Port=2
  Action Port : ActionPort  ActionType=else
  Constant : Constant  Value=PHAONTISUMMAX_NANOSEC_U32
  CopyRight1 : Subsystem  Description=|  mask(Copyright Information){none=on}
      | Copyright info block.                                               
      |                                                                     
      | Place copyright information at the top of every subsystem in design.
      mask prompts: none "No parameters"
      mask help: Place copyright information at the top of every subsystem in design.
      mask Display:
      | NxtrConf = 'Nexteer Confidential';
      | 
      | sys = bdroot; %handle for the current model ("system")
      | first = get_param(sys,'Created');
      | first = first(end-3:end);  %year is last four digits
      | 
      | last = get_param(sys,'LastModifiedDate');
      | if isempty(last)
      |     last = datestr(now,'yyyy');
      | else
      |     last = last(end-3:end);
      | end
      | 
      | if strcmp(first,last)
      |     fprintf('%s -- Copyright %s Nexteer',NxtrConf,first)
      | else
      |     fprintf('%s -- %s%s- %s Nexteer',NxtrConf,char(169),first,last)
      | end
  Sum : Sum  Inputs=++-  OutDataTypeStr=uint32
  PhaOnTiSumAExp : Outport
  wires:
  Sum/1 -> PhaOnTiSumAExp/1
  PhaOnTiSumA/1 -> Sum/2
  Constant/1 -> Sum/1
  MotDrvDiagcPhaOnTiSumAPrev/1 -> Sum/3

== system ES320A_MotDrvDiagc/MotDrvDiagc/MotDrvDiagcPer1/DeltaCompu/else1 ==
  PhaOnTiSumB : Inport
  MotDrvDiagcPhaOnTiSumBPrev : Inport  Port=2
  Action Port : ActionPort  ActionType=else
  Constant : Constant  Value=PHAONTISUMMAX_NANOSEC_U32
  CopyRight1 : Subsystem  Description=|  mask(Copyright Information){none=on}
      | Copyright info block.                                               
      |                                                                     
      | Place copyright information at the top of every subsystem in design.
      mask prompts: none "No parameters"
      mask help: Place copyright information at the top of every subsystem in design.
      mask Display:
      | NxtrConf = 'Nexteer Confidential';
      | 
      | sys = bdroot; %handle for the current model ("system")
      | first = get_param(sys,'Created');
      | first = first(end-3:end);  %year is last four digits
      | 
      | last = get_param(sys,'LastModifiedDate');
      | if isempty(last)
      |     last = datestr(now,'yyyy');
      | else
      |     last = last(end-3:end);
      | end
      | 
      | if strcmp(first,last)
      |     fprintf('%s -- Copyright %s Nexteer',NxtrConf,first)
      | else
      |     fprintf('%s -- %s%s- %s Nexteer',NxtrConf,char(169),first,last)
      | end
  Sum : Sum  Inputs=++-  OutDataTypeStr=uint32
  PhaOnTiSumBExp : Outport
  wires:
  Sum/1 -> PhaOnTiSumBExp/1
  PhaOnTiSumB/1 -> Sum/2
  Constant/1 -> Sum/1
  MotDrvDiagcPhaOnTiSumBPrev/1 -> Sum/3

== system ES320A_MotDrvDiagc/MotDrvDiagc/MotDrvDiagcPer1/DeltaCompu/else2 ==
  PhaOnTiSumC : Inport
  MotDrvDiagcPhaOnTiSumCPrev : Inport  Port=2
  Action Port : ActionPort  ActionType=else
  Constant : Constant  Value=PHAONTISUMMAX_NANOSEC_U32
  CopyRight1 : Subsystem  Description=|  mask(Copyright Information){none=on}
      | Copyright info block.                                               
      |                                                                     
      | Place copyright information at the top of every subsystem in design.
      mask prompts: none "No parameters"
      mask help: Place copyright information at the top of every subsystem in design.
      mask Display:
      | NxtrConf = 'Nexteer Confidential';
      | 
      | sys = bdroot; %handle for the current model ("system")
      | first = get_param(sys,'Created');
      | first = first(end-3:end);  %year is last four digits
      | 
      | last = get_param(sys,'LastModifiedDate');
      | if isempty(last)
      |     last = datestr(now,'yyyy');
      | else
      |     last = last(end-3:end);
      | end
      | 
      | if strcmp(first,last)
      |     fprintf('%s -- Copyright %s Nexteer',NxtrConf,first)
      | else
      |     fprintf('%s -- %s%s- %s Nexteer',NxtrConf,char(169),first,last)
      | end
  Sum : Sum  Inputs=++-  OutDataTypeStr=uint32
  PhaOnTiSumCExp : Outport
  wires:
  Sum/1 -> PhaOnTiSumCExp/1
  PhaOnTiSumC/1 -> Sum/2
  Constant/1 -> Sum/1
  MotDrvDiagcPhaOnTiSumCPrev/1 -> Sum/3

== system ES320A_MotDrvDiagc/MotDrvDiagc/MotDrvDiagcPer1/DeltaCompu/if ==
  PhaOnTiSumA : Inport
  MotDrvDiagcPhaOnTiSumAPrev : Inport  Port=2
  Action Port : ActionPort  ActionType=then
  CopyRight1 : Subsystem  Description=|  mask(Copyright Information){none=on}
      | Copyright info block.                                               
      |                                                                     
      | Place copyright information at the top of every subsystem in design.
      mask prompts: none "No parameters"
      mask help: Place copyright information at the top of every subsystem in design.
      mask Display:
      | NxtrConf = 'Nexteer Confidential';
      | 
      | sys = bdroot; %handle for the current model ("system")
      | first = get_param(sys,'Created');
      | first = first(end-3:end);  %year is last four digits
      | 
      | last = get_param(sys,'LastModifiedDate');
      | if isempty(last)
      |     last = datestr(now,'yyyy');
      | else
      |     last = last(end-3:end);
      | end
      | 
      | if strcmp(first,last)
      |     fprintf('%s -- Copyright %s Nexteer',NxtrConf,first)
      | else
      |     fprintf('%s -- %s%s- %s Nexteer',NxtrConf,char(169),first,last)
      | end
  Sum : Sum  Inputs=|+-  OutDataTypeStr=uint32
  PhaOnTiSumAExp : Outport
  wires:
  Sum/1 -> PhaOnTiSumAExp/1
  PhaOnTiSumA/1 -> Sum/1
  MotDrvDiagcPhaOnTiSumAPrev/1 -> Sum/2

== system ES320A_MotDrvDiagc/MotDrvDiagc/MotDrvDiagcPer1/DeltaCompu/if1 ==
  PhaOnTiSumB : Inport
  MotDrvDiagcPhaOnTiSumBPrev : Inport  Port=2
  Action Port : ActionPort  ActionType=then
  CopyRight1 : Subsystem  Description=|  mask(Copyright Information){none=on}
      | Copyright info block.                                               
      |                                                                     
      | Place copyright information at the top of every subsystem in design.
      mask prompts: none "No parameters"
      mask help: Place copyright information at the top of every subsystem in design.
      mask Display:
      | NxtrConf = 'Nexteer Confidential';
      | 
      | sys = bdroot; %handle for the current model ("system")
      | first = get_param(sys,'Created');
      | first = first(end-3:end);  %year is last four digits
      | 
      | last = get_param(sys,'LastModifiedDate');
      | if isempty(last)
      |     last = datestr(now,'yyyy');
      | else
      |     last = last(end-3:end);
      | end
      | 
      | if strcmp(first,last)
      |     fprintf('%s -- Copyright %s Nexteer',NxtrConf,first)
      | else
      |     fprintf('%s -- %s%s- %s Nexteer',NxtrConf,char(169),first,last)
      | end
  Sum : Sum  Inputs=|+-  OutDataTypeStr=uint32
  PhaOnTiSumBExp : Outport
  wires:
  Sum/1 -> PhaOnTiSumBExp/1
  PhaOnTiSumB/1 -> Sum/1
  MotDrvDiagcPhaOnTiSumBPrev/1 -> Sum/2

== system ES320A_MotDrvDiagc/MotDrvDiagc/MotDrvDiagcPer1/DeltaCompu/if2 ==
  PhaOnTiSumC : Inport
  MotDrvDiagcPhaOnTiSumCPrev : Inport  Port=2
  Action Port : ActionPort  ActionType=then
  CopyRight1 : Subsystem  Description=|  mask(Copyright Information){none=on}
      | Copyright info block.                                               
      |                                                                     
      | Place copyright information at the top of every subsystem in design.
      mask prompts: none "No parameters"
      mask help: Place copyright information at the top of every subsystem in design.
      mask Display:
      | NxtrConf = 'Nexteer Confidential';
      | 
      | sys = bdroot; %handle for the current model ("system")
      | first = get_param(sys,'Created');
      | first = first(end-3:end);  %year is last four digits
      | 
      | last = get_param(sys,'LastModifiedDate');
      | if isempty(last)
      |     last = datestr(now,'yyyy');
      | else
      |     last = last(end-3:end);
      | end
      | 
      | if strcmp(first,last)
      |     fprintf('%s -- Copyright %s Nexteer',NxtrConf,first)
      | else
      |     fprintf('%s -- %s%s- %s Nexteer',NxtrConf,char(169),first,last)
      | end
  Sum : Sum  Inputs=|+-  OutDataTypeStr=uint32
  PhaOnTiSumCExp : Outport
  wires:
  Sum/1 -> PhaOnTiSumCExp/1
  PhaOnTiSumC/1 -> Sum/1
  MotDrvDiagcPhaOnTiSumCPrev/1 -> Sum/2

== system ES320A_MotDrvDiagc/MotDrvDiagc/MotDrvDiagcPer1/MotDrvDiagcFltChk/Copyright1 ==

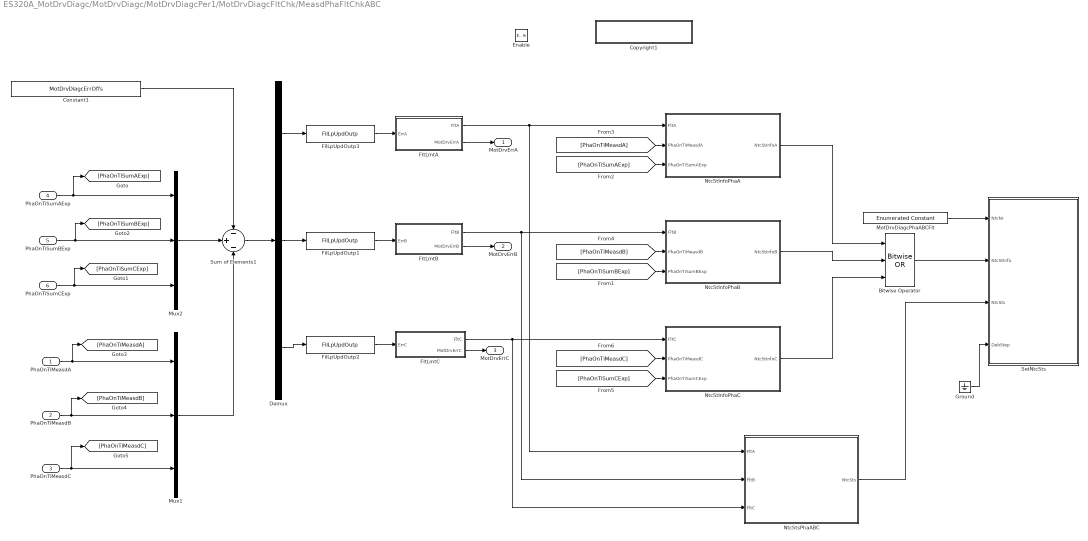
== system ES320A_MotDrvDiagc/MotDrvDiagc/MotDrvDiagcPer1/MotDrvDiagcFltChk/MeasdPhaFltChkABC ==
  PhaOnTiMeasdA : Inport
  PhaOnTiMeasdB : Inport  Port=2
  PhaOnTiMeasdC : Inport  Port=3
  PhaOnTiSumAExp : Inport  Port=4
  PhaOnTiSumBExp : Inport  Port=5
  PhaOnTiSumCExp : Inport  Port=6
  Enable : EnablePort  StatesWhenEnabling=reset
  Bitwise Operator : simulink/Logic and Bit Operations/Bitwise Operator  logicop=OR  UseBitMask=off  NumInputPorts=3  BitMask=bin2dec('11011001')  BitMaskRealWorld=Stored Integer
  Constant1 : Constant  Value=MotDrvDiagcErrOffs
  Copyright1 : Subsystem  Description=|  RequirementInfo={} %GIDa_3494648b_2e9c_42f3_92a1_ee669197cb15  mask(Copyright Information){none=on}
      | Copyright info block.                                               
      |                                                                     
      | Place copyright information at the top of every subsystem in design.
      mask prompts: none "No parameters"
      mask help: Place copyright information at the top of every subsystem in design.
      mask Display:
      | NxtrConf = 'Nexteer Confidential';
      | 
      | sys = bdroot; %handle for the current model ("system")
      | first = get_param(sys,'Created');
      | if(isempty(first))
      |     first = datestr(now,'yyyy');
      | else
      |     first = first(end-3:end);  %year is last four digits
      | end
      | 
      | last = get_param(sys,'LastModifiedDate');
      | if isempty(last)
      |     last = datestr(now,'yyyy');
      | else
      |     last = last(end-3:end);
      | end
      | 
      | if strcmp(first,last)
      |     fprintf('%s\nCopyright  %s Nexteer',NxtrConf,first);
      | else
      |     fprintf('%s\n%s%s-%s Nexteer',NxtrConf,char(169),first,last);
      | end
  Demux : Demux  Outputs=3
  FilLpUpdOutp1 : Fil/FilLpUpdOutp  StVar=MotDrvDiagcPhaBFilLp
      settings: AttributesFormatString=StVar: %<StVar>
  FilLpUpdOutp2 : Fil/FilLpUpdOutp  StVar=MotDrvDiagcPhaCFilLp
      settings: AttributesFormatString=StVar: %<StVar>
  FilLpUpdOutp3 : Fil/FilLpUpdOutp  StVar=MotDrvDiagcPhaAFilLp
      settings: AttributesFormatString=StVar: %<StVar>
  FltLmtA : Subsystem  RequirementInfo={'linktype_rmi_doors' '0000cf4c (/ESG Group/FDD Module Requirements/EA4 Specific/ES320A_MotDrvDiagc)' '#ES320A_209' 'true' 'REQ: ES320A_209' '' } %GIDa_24cbd451_4da8_4119_bffb_040324b5d539
  FltLmtB : Subsystem  RequirementInfo={'linktype_rmi_doors' '0000cf4c (/ESG Group/FDD Module Requirements/EA4 Specific/ES320A_MotDrvDiagc)' '#ES320A_214' 'true' 'REQ: ES320A_214' '' } %GIDa_1a18998f_b18b_499f_8985_82b7072e45d0
  FltLmtC : Subsystem  RequirementInfo={'linktype_rmi_doors' '0000cf4c (/ESG Group/FDD Module Requirements/EA4 Specific/ES320A_MotDrvDiagc)' '#ES320A_213' 'true' 'REQ: ES320A_213' '' } %GIDa_a2352b55_c282_42fc_bf6a_022c54caeb36
  Ground : Ground
  MotDrvDiagcPhaABCFlt : simulink/Sources/Enumerated Constant  OutDataTypeStr=Enum: NtcNr1  Value=NtcNr1.NTCNR_0X054  SampleTime=inf
  Mux1 : Mux  Inputs=3
  Mux2 : Mux  Inputs=3
  NtcStInfoPhaA : Subsystem
  NtcStInfoPhaB : Subsystem
  NtcStInfoPhaC : Subsystem
  NtcStsPhaABC : Subsystem  RequirementInfo={'linktype_rmi_doors' '0000cf4c (/ESG Group/FDD Module Requirements/EA4 Specific/ES320A_MotDrvDiagc)' '#ES320A_202' 'true' 'REQ: ES320A_202' '' } %GIDa_d834093a_8cc1_494c_9266_09ccb87f0544
  SetNtcSts : Subsystem  RequirementInfo={'linktype_rmi_doors' '0000cf4c (/ESG Group/FDD Module Requirements/EA4 Specific/ES320A_MotDrvDiagc)' '#ES320A_157' 'true' 'REQ: ES320A_157' '' } %GIDa_1403571e_c02b_42b7_b7b5_e1dfc1b60447
  Sum of Elements1 : Sum  Inputs=-+-  OutDataTypeStr=single
  MotDrvErrA : Outport
  MotDrvErrB : Outport  Port=2
  MotDrvErrC : Outport  Port=3
  wires:
  MotDrvDiagcPhaABCFlt/1 -> SetNtcSts/1(NtcNr)
  FltLmtA/1(FltA) -> NtcStsPhaABC/1(FltA), NtcStInfoPhaA/1(FltA)
  FltLmtB/1(FltB) -> NtcStsPhaABC/2(FltB), NtcStInfoPhaB/1(FltB)
  FltLmtC/1(FltC) -> NtcStsPhaABC/3(FltC), NtcStInfoPhaC/1(FltC)
  [PhaOnTiSumAExp] -> NtcStInfoPhaA/3(PhaOnTiSumAExp)
  [PhaOnTiMeasdB] -> NtcStInfoPhaB/2(PhaOnTiMeasdB)
  [PhaOnTiSumBExp] -> NtcStInfoPhaB/3(PhaOnTiSumBExp)
  [PhaOnTiMeasdC] -> NtcStInfoPhaC/2(PhaOnTiMeasdC)
  [PhaOnTiSumCExp] -> NtcStInfoPhaC/3(PhaOnTiSumCExp)
  NtcStInfoPhaA/1(NtcStInfoA) -> Bitwise Operator/1
  NtcStInfoPhaB/1(NtcStInfoB) -> Bitwise Operator/2
  NtcStInfoPhaC/1(NtcStInfoC) -> Bitwise Operator/3
  NtcStsPhaABC/1(NtcSts) -> SetNtcSts/3(NtcSts)
  Demux/1 -> FilLpUpdOutp3/1
  Demux/2 -> FilLpUpdOutp1/1
  Demux/3 -> FilLpUpdOutp2/1
  FilLpUpdOutp3/1 -> FltLmtA/1(ErrA)
  FilLpUpdOutp1/1 -> FltLmtB/1(ErrB)
  FilLpUpdOutp2/1 -> FltLmtC/1(ErrC)
  [PhaOnTiMeasdA] -> NtcStInfoPhaA/2(PhaOnTiMeasdA)
  Bitwise Operator/1 -> SetNtcSts/2(NtcStInfo)
  Ground/1 -> SetNtcSts/4(DebStep)
  PhaOnTiMeasdB/1 -> [PhaOnTiMeasdB], Mux1/2
  PhaOnTiMeasdC/1 -> [PhaOnTiMeasdC], Mux1/3
  PhaOnTiMeasdA/1 -> [PhaOnTiMeasdA], Mux1/1
  Sum of Elements1/1 -> Demux/1
  Constant1/1 -> Sum of Elements1/1
  Mux1/1 -> Sum of Elements1/3
  Mux2/1 -> Sum of Elements1/2
  PhaOnTiSumAExp/1 -> [PhaOnTiSumAExp], Mux2/1
  PhaOnTiSumBExp/1 -> [PhaOnTiSumBExp], Mux2/2
  PhaOnTiSumCExp/1 -> [PhaOnTiSumCExp], Mux2/3
  FltLmtA/2(MotDrvErrA) -> MotDrvErrA/1
  FltLmtB/2(MotDrvErrB) -> MotDrvErrB/1
  FltLmtC/2(MotDrvErrC) -> MotDrvErrC/1
